simulink model "PRACTICE_1"  (R2021b)
settings: Solver=VariableStepAuto  StartTime=0.0  StopTime=0.01  RelTol=1e-3
undefined symbols (not defined in the file): magnitude
libraries: dsparch4 x1
settings Model: Creator=Joshua  LastModifiedBy=Joshua

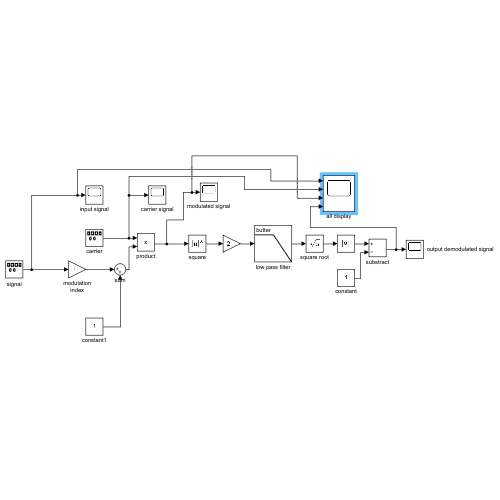
[thumbnail: Simulink's stored preview of the top-level diagram]
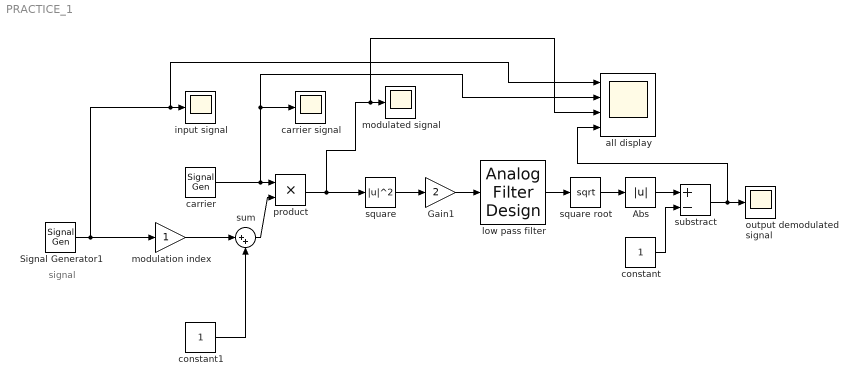
== system PRACTICE_1 ==
  note: signal
  Abs : Abs
  Gain1 : Gain  Gain=2
  Signal Generator1 : SignalGenerator  Frequency=1000
  all display : Scope  NumInputPorts=4
  carrier : SignalGenerator  Frequency=20000
  carrier signal : Scope
  constant : Constant
  constant1 : Constant
  input signal : Scope
  low pass filter : dsparch4/Analog Filter Design  method=Butterworth  filttype=Lowpass  N=8  Wlo=2*pi*11000  Whi=80  Rp=2  Rs=40
  modulated signal : Scope
  modulation index : Gain
  output demodulated signal : Scope
  product : Product
  square : Math  Operator=magnitude^2  SaturateOnIntegerOverflow=on
  square root : Sqrt  SaturateOnIntegerOverflow=on
  substract : Sum  Inputs=+-
  sum : Sum  Inputs=|++
  wires:
  constant1/1 -> sum/2
  sum/1 -> product/2
  carrier/1 -> all display/2, carrier signal/1, product/1
  square/1 -> Gain1/1
  product/1 -> all display/3, modulated signal/1, square/1
  Gain1/1 -> low pass filter/1
  low pass filter/1 -> square root/1
  square root/1 -> Abs/1
  Abs/1 -> substract/1
  substract/1 -> all display/4, output demodulated signal/1
  constant/1 -> substract/2
  modulation index/1 -> sum/1
  Signal Generator1/1 -> all display/1, input signal/1, modulation index/1
